simulink model "singlePhasePWMrectifierOpen"  (R2019b)
settings: Solver=ode23  StartTime=0.0  StopTime=5  RelTol=1e-3
libraries: powerlib x17, simulink x1
settings Model: SimulationMode=accelerator  Creator=YJP  LastModifiedBy=YJP
settings SolverCC: ZeroCrossAlgorithm=Adaptive
settings DataIOCC: SaveFormat=StructureWithTime  ReturnWorkspaceOutputs=off
settings OptimizationCC: LifeSpan=inf
settings DebuggingCC: IgnoredZcDiagnostic=none  SFExecutionAtInitializationDiag=none  ArithmeticOperatorsInVariantConditions=warning
settings HardwareCC: ProdBitPerSizeT=32  ProdBitPerPtrDiffT=32  ProdWordSize=32  ProdHWDeviceType=Specified
settings SFSimCC: CustomCodeUndefinedFunction=UseInterfaceOnly
settings CodeAppCC: StateflowObjectComments=on

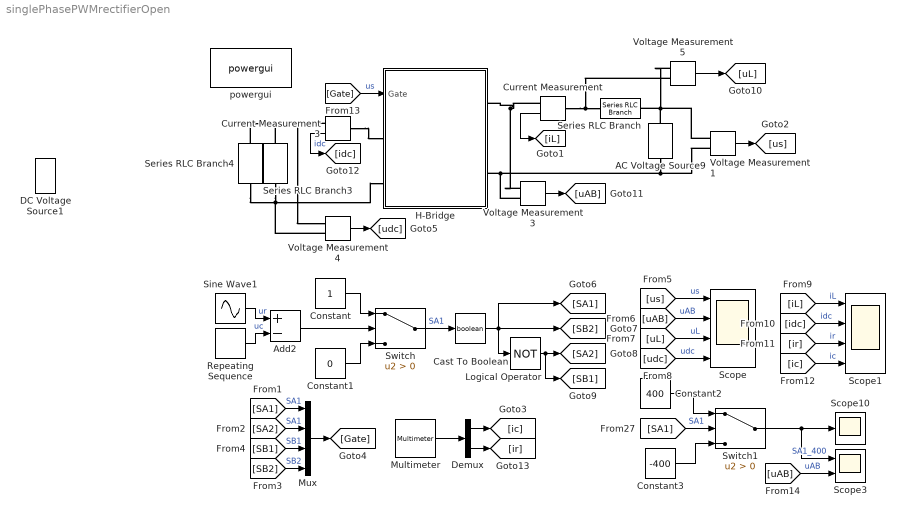
== system singlePhasePWMrectifierOpen ==
  AC Voltage Source9 : powerlib/Electrical Sources/AC Voltage Source  Amplitude=250  Phase=-38  Frequency=50  SampleTime=0  Measurements=None  BusType=swing  Pref=10e3  Qref=0  Qmin=-inf  Qmax=+inf
      settings: SourceProductName=Simscape Electrical
  Add2 : Sum  Inputs=+-
  Cast To Boolean : DataTypeConversion  OutDataTypeStr=boolean
  Constant : Constant
  Constant1 : Constant  Value=0
  Constant2 : Constant  Value=400
  Constant3 : Constant  Value=-400
  Current Measurement : powerlib/Measurements/Current Measurement  PhasorSimulation=off  OutputType=Complex  PSBequivalent=0
      settings: SourceProductName=Simscape Electrical
  Current Measurement3 : powerlib/Measurements/Current Measurement  PhasorSimulation=off  OutputType=Complex  PSBequivalent=0
      settings: SourceProductName=Simscape Electrical
  DC Voltage Source1 : powerlib/Electrical Sources/DC Voltage Source  Amplitude=420  Measurements=None
      settings: SourceProductName=Simscape Electrical
  Demux : Demux  Outputs=2
  H-Bridge : Subsystem
  Logical Operator : Logic  Operator=NOT  AllPortsSameDT=off  OutDataTypeStr=boolean
  Multimeter : powerlib/Measurements/Multimeter  PhasorSimulation=off  OutputType=Complex  sel=[1 2]  L=2  Gain=[1 1]  yselected={'Ib: Series RLC Branch3','Ib: Series RLC Branch4'};  PSBOutputType=1  PSBequivalent=0  AxesSetting=[0,0.1,-100,100]  Display=0  SavedBlockNames=-11
      settings: SourceProductName=Simscape Electrical
  Mux : Mux
  Repeating Sequence : simulink/Sources/Repeating Sequence  rep_seq_t=[0 5e-5 10e-5]  rep_seq_y=[-1 1 -1]
  Scope : Scope  NumInputPorts=4
  Scope1 : Scope  NumInputPorts=4
  Scope10 : Scope
  Scope3 : Scope  NumInputPorts=2
  Series RLC Branch : powerlib/Elements/Series RLC Branch  LConnTagsString=__new0  RConnTagsString=__new0  BranchType=RL  Resistance=1e-1  Inductance=5e-3  SetiL0=off  InitialCurrent=0  Capacitance=1e-6  Setx0=off  InitialVoltage=0  Measurements=None
      settings: SourceProductName=Simscape Electrical
  Series RLC Branch3 : powerlib/Elements/Series RLC Branch  LConnTagsString=__new0  RConnTagsString=__new0  BranchType=C  Resistance=10  Inductance=1e-3  SetiL0=off  InitialCurrent=0  Capacitance=1e-3  Setx0=off  InitialVoltage=0  Measurements=Branch current
      settings: SourceProductName=Simscape Electrical
  Series RLC Branch4 : powerlib/Elements/Series RLC Branch  LConnTagsString=__new0  RConnTagsString=__new0  BranchType=R  Resistance=44.117  Inductance=1e-3  SetiL0=off  InitialCurrent=0  Capacitance=10e-6  Setx0=off  InitialVoltage=0  Measurements=Branch current
      settings: SourceProductName=Simscape Electrical
  Sine Wave1 : Sin  Amplitude=0.54  Frequency=100*pi  Phase=-0.28111*pi  SampleTime=0
  Switch : Switch  Criteria=u2 > Threshold
  Switch1 : Switch  Criteria=u2 > Threshold
  Voltage Measurement{1,3..5} (4 alike) : powerlib/Measurements/Voltage Measurement  PhasorSimulation=off  OutputType=Complex  PSBequivalent=0
      settings: SourceProductName=Simscape Electrical
  powergui : powerlib/powergui  Priority=1  SimulationMode=Discrete  SampleTime=1e-6  frequency=60  Iterations=50  frequencyindice=0  Pbase=100e6  ErrMax=1e-4  UnitsV=kV  UnitsW=MW  buscounter=0  FunctionMessages=off  echomessages=off  EnableUseOfTLC=off  CurrentSourceSwitches=off  DisableSnubberDevices=off  DisableRonSwitches=off  DisableVfSwitches=off  DisplayEquations=off  AutomaticDiscreteSolvers=off  SolverType=Tustin/Backward Euler (TBE)  Interpol=off  ExternalGateDelay=off  methode=off  Ts=100  x0status=blocks  SPID=on  SwTol=0  HookPort=off  NonlinearTolerance=1e-4  nMaxIteration=100  ContinueOnMaxIteration=off  RestoreLinks=warning  ResistiveCurrentMeasurement=off  Frange=[0:2:500]  Ylog=off  Xlog=on  ShowGrid=off  save=off  variable=ZData  structure=SA1_400  ZoomFFT=off  StartTime=0.1  cycles=2  DisplayStyle=4  fundamental=50  FreqAxis=off  MaxFrequency=12000  frequencyindicesteady=1  RmsSteady=1  display=off
      settings: SourceProductName=Simscape Electrical
  wires:
  Repeating Sequence/1 -> Add2/2  "uc"
  Add2/1 -> Switch/2
  Constant/1 -> Switch/1
  Constant1/1 -> Switch/3
  Switch/1 -> Cast To Boolean/1  "SA1"
  Logical Operator/1 -> [SA2], [SB1]
  Voltage Measurement3/1 -> [uAB]
  Sine Wave1/1 -> Add2/1  "ur"
  [SA1] -> Mux/1  "SA1"
  [SA2] -> Mux/2  "SA1"
  [SB2] -> Mux/4  "SB2"
  [SB1] -> Mux/3  "SB1"
  Mux/1 -> [Gate]
  Voltage Measurement4/1 -> [udc]
  Current Measurement3/1 -> [idc]  "idc"
  Current Measurement/1 -> [iL]
  Voltage Measurement1/1 -> [us]
  Voltage Measurement5/1 -> [uL]
  Constant3/1 -> Switch1/3
  Constant2/1 -> Switch1/1
  Switch1/1 -> Scope3/1, Scope10/1  "SA1_400"
  [SA1] -> Switch1/2  "SA1"
  [us] -> Scope/1  "us"
  [uAB] -> Scope/2  "uAB"
  [uL] -> Scope/3  "uL"
  [udc] -> Scope/4  "udc"
  [iL] -> Scope1/1  "iL"
  [idc] -> Scope1/2  "idc"
  Multimeter/1 -> Demux/1
  Demux/1 -> [ic]
  Demux/2 -> [ir]
  [ir] -> Scope1/3  "ir"
  [ic] -> Scope1/4  "ic"
  Cast To Boolean/1 -> [SA1], Logical Operator/1, [SB2]
  [Gate] -> H-Bridge/1(Gate)  "us"
  [uAB] -> Scope3/2  "uAB"
  connections:
  AC Voltage Source9/RConn1 -- Voltage Measurement1/LConn1 -- Voltage Measurement5/LConn1 -- Series RLC Branch/RConn1
  Series RLC Branch4/RConn1 -- Voltage Measurement4/LConn2 -- H-Bridge/LConn2 -- Series RLC Branch3/RConn1
  Current Measurement3/LConn1 -- H-Bridge/LConn1
  Current Measurement3/RConn1 -- Series RLC Branch4/LConn1 -- Series RLC Branch3/LConn1 -- Voltage Measurement4/LConn1
  AC Voltage Source9/LConn1 -- Voltage Measurement3/LConn2 -- H-Bridge/RConn2 -- Voltage Measurement1/LConn2
  Current Measurement/LConn1 -- Voltage Measurement5/LConn2 -- Series RLC Branch/LConn1
  Current Measurement/RConn1 -- Voltage Measurement3/LConn1 -- H-Bridge/RConn1

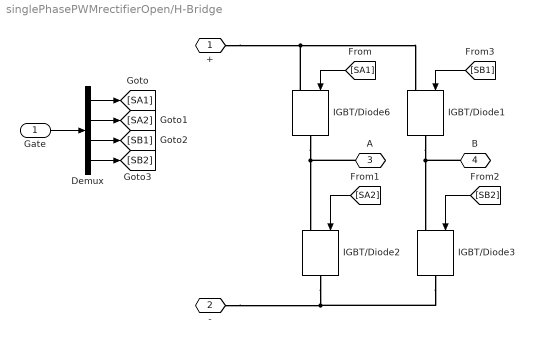
== system singlePhasePWMrectifierOpen/H-Bridge ==
  Gate : Inport
  Demux : Demux
  IGBT/Diode{1..3,6} (4 alike) : powerlib/Power Electronics/IGBT//Diode  Ron=1e-3  Rs=1e5  Cs=inf  Measurements=off
      settings: SourceProductName=Simscape Electrical
  + : PMIOPort  Side=Left
  - : PMIOPort  Port=2  Side=Left
  A : PMIOPort  Port=3  Side=Right
  B : PMIOPort  Port=4  Side=Right
  wires:
  [SA1] -> IGBT/Diode6/1
  [SB1] -> IGBT/Diode1/1
  [SA2] -> IGBT/Diode2/1
  [SB2] -> IGBT/Diode3/1
  Demux/1 -> [SA1]
  Demux/2 -> [SA2]
  Demux/3 -> [SB1]
  Demux/4 -> [SB2]
  Gate/1 -> Demux/1
  connections:
  IGBT/Diode1/RConn1 -- B/RConn1 -- IGBT/Diode3/LConn1
  IGBT/Diode6/LConn1 -- +/RConn1 -- IGBT/Diode1/LConn1
  IGBT/Diode6/RConn1 -- A/RConn1 -- IGBT/Diode2/LConn1
  IGBT/Diode3/RConn1 -- -/RConn1 -- IGBT/Diode2/RConn1
